simulink model "ett_slap"  (R2014b)
settings: Solver=ode45  SolverMode=SingleTasking  StartTime=0.0  StopTime=500  RelTol=1e-3
values from neighbouring files (symbols this model uses):
  Xd = [phi1e]    [ett_slap.m]    (also in linearss_circle.m = [phi3e;phi2e;phi1e]; tva_slap.m = [phi2e;phi1e])
undefined symbols (not defined in the file or in its folder): K
libraries: simulink x4, simulink_extras x3
settings Model: Creator=marcus  LastModifiedBy=marcus
settings OptimizationCC: BlockReduction=off  BooleanDataType=off  UseDivisionForNetSlopeComputation=off  SimCompilerOptimization=off
settings DebuggingCC: SaveWithParameterizedLinksMsg=none  UnderspecifiedInitializationDetection=Classic  MergeDetectMultiDrivingBlocksExec=none  SignalResolutionControl=TryResolveAllWithWarning  SolverPrmCheckMsg=none  FrameProcessingCompatibilityMsg=error
settings HardwareCC: TargetUnknown=on
settings RTWCC: RTWCompilerOptimization=off

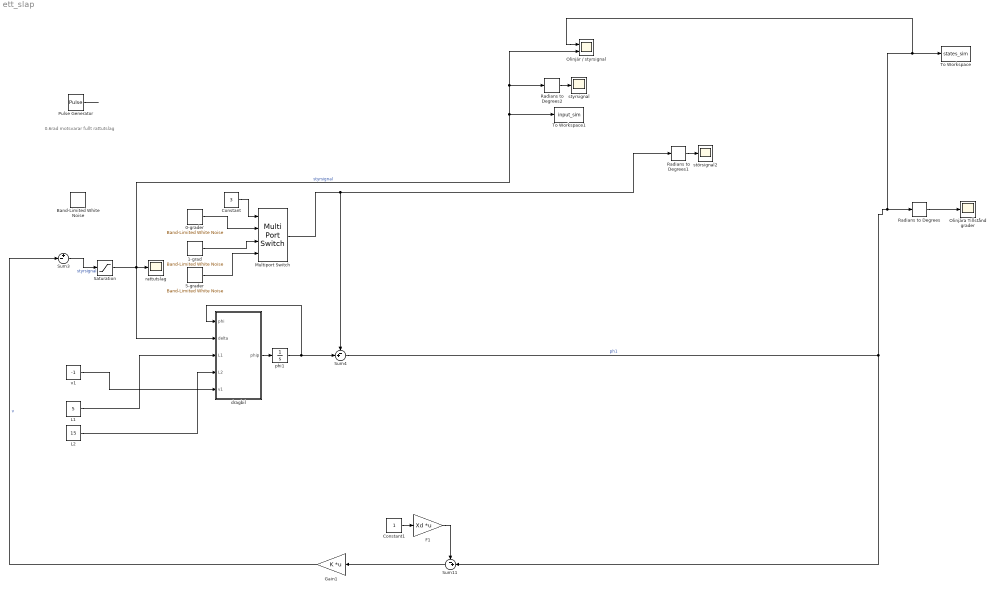
== system ett_slap ==
  note: 0.6rad motsvarar fullt rattutslag
  0-grader : simulink/Sources/Band-Limited White Noise  Cov=[0.00000]  Ts=0.1  seed=[1]
  1-grad : simulink/Sources/Band-Limited White Noise  Cov=[0.000005]  Ts=0.1  seed=[1]
  5-grader : simulink/Sources/Band-Limited White Noise  Cov=[0.00009]  Ts=0.1  seed=[1]
  Band-Limited White Noise : simulink/Sources/Band-Limited White Noise  Cov=[0.0001]  Ts=0.1  seed=[23341]
  Constant : Constant  Value=3  VectorParams1D=off  SampleTime=-1
  Constant1 : Constant
  F1 : Gain  Gain=Xd  Multiplication=Matrix(K*u)
  Gain1 : Gain  Gain=K  Multiplication=Matrix(K*u)
  L1 : Constant  Value=5  SampleTime=1
  L2 : Constant  Value=15  SampleTime=1
  Multiport Switch : MultiPortSwitch
  Olinjär / styrsignal : Scope  NumInputPorts=2
      settings: TickLabels=on  ShowLegends=on  YMin=-5~-0.2  YMax=2~0.4
  Olinjära Tillstånd grader : Scope
      settings: ShowLegends=on
  Pulse Generator : DiscretePulseGenerator  PulseType=Time based  Amplitude=0.1  Period=1000  PhaseDelay=5
  Radians to Degrees : simulink_extras/Transformations/Radians to Degrees
  Radians to Degrees1 : simulink_extras/Transformations/Radians to Degrees
  Radians to Degrees2 : simulink_extras/Transformations/Radians to Degrees
  Saturation : Saturate  UpperLimit=0.7  LowerLimit=-0.7
  Sum11 : Sum  Inputs=-+|
  Sum3 : Sum  Inputs=+-|
  Sum4 : Sum  Inputs=-+|
  To Workspace : ToWorkspace  VariableName=states_sim  SampleTime=-1
      settings: Save2DSignal=2-D array (concatenate along first dimension)
  To Workspace1 : ToWorkspace  VariableName=input_sim  SampleTime=-1
      settings: Save2DSignal=2-D array (concatenate along first dimension)
  dragbil : MATLAB Function  TreatAsAtomicUnit=on
  phi1 : Integrator
  rattutslag : Scope
      settings: ShowLegends=on  SaveName=ScopeData2
  styrsignal : Scope
      settings: ShowLegends=on  SaveName=ScopeData6
  störsignal2 : Scope
      settings: ShowLegends=on  SaveName=ScopeData5
  v1 : Constant  Value=-1  SampleTime=1
  wires:
  dragbil/1(phip) -> phi1/1
  v1/1 -> dragbil/5(v1)
  L2/1 -> dragbil/4(L2)
  L1/1 -> dragbil/3(L1)
  Gain1/1 -> Sum3/2  "v"
  Multiport Switch/1 -> Radians to Degrees1/1, Sum4/1
  Sum4/1 -> Olinjär / styrsignal/1, To Workspace/1, Radians to Degrees/1, Sum11/2  "ph1"
  Saturation/1 -> rattutslag/1, To Workspace1/1, Olinjär / styrsignal/2, Radians to Degrees2/1, dragbil/2(delta)  "styrsignal"
  Pulse Generator/1 -> ?
  phi1/1 -> Sum4/2, dragbil/1(phi)
  Sum11/1 -> Gain1/1
  Constant1/1 -> F1/1
  Radians to Degrees/1 -> Olinjära Tillstånd grader/1
  Radians to Degrees1/1 -> störsignal2/1
  Radians to Degrees2/1 -> styrsignal/1
  Sum3/1 -> Saturation/1  "styrsignal"
  F1/1 -> Sum11/1
  0-grader/1 -> Multiport Switch/2
  5-grader/1 -> Multiport Switch/4
  1-grad/1 -> Multiport Switch/3
  Constant/1 -> Multiport Switch/1

== matlab function ett_slap/dragbil ==
  data: phi input; delta input; phip output; L1 input; L2 input; v1 input
function phip = fcn(phi,delta,L1,L2,v1)
%#codegen

phip = v1*(tan(delta)/L1-sin(phi)/L2);
